simulink model "platform"  (R2020a)
settings: Solver=VariableStepAuto  StartTime=0.0  StopTime=10.0  RelTol=1e-3
undefined symbols (not defined in the file): R
settings Model: Creator=daixingze  LastModifiedBy=daixingze

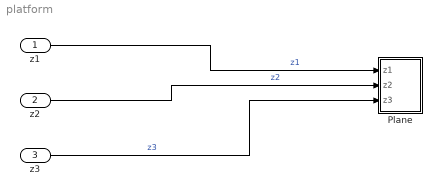
== system platform ==
  z1 : Inport
  z2 : Inport  Port=2
  z3 : Inport  Port=3
  Plane : Subsystem
  wires:
  z1/1 -> Plane/1(z1)  "z1"
  z2/1 -> Plane/2(z2)  "z2"
  z3/1 -> Plane/3(z3)  "z3"

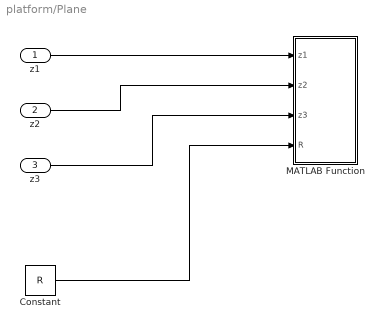
== system platform/Plane ==
  z1 : Inport
  z2 : Inport  Port=2
  z3 : Inport  Port=3
  Constant : Constant  Value=R
  MATLAB Function : MATLAB Function  TreatAsAtomicUnit=on
  wires:
  z3/1 -> MATLAB Function/3(z3)
  z1/1 -> MATLAB Function/1(z1)
  z2/1 -> MATLAB Function/2(z2)
  Constant/1 -> MATLAB Function/4(R)

== matlab function platform/Plane/MATLAB Function ==
  data: z1 input; z2 input; z3 input; R input
function fcn(z1,z2,z3,R)
    % Linear servo position on the plane.
    o1 = [1,0];
    o2 = [-1/2, sqrt(3)/2];
    o3 = [-1/2, -sqrt(3)/2];
    
    % prismatic position
    p1 = [o1*R, z1];
    p2 = [o2*R, z2];
    p3 = [o3*R, z3];
    
%     % plane vector
%     t1 = p2-p1;
%     t2 = p3-p1;
    
    % Draw plane
    x = [p1(1),p2(1),p3(1)];
    y = [p1(2),p2(2),p3(2)];
    z = [z1, z2, z3];
%     figure;
%     plot3(x,y,z);
